simulink model "ControllerDesign_Lon"  (R2017b)
settings: Solver=VariableStepAuto  StartTime=0.0  StopTime=5  RelTol=1e-3
undefined symbols (not defined in the file or in its folder): Linmod
settings Model: Creator=One  LastModifiedBy=One

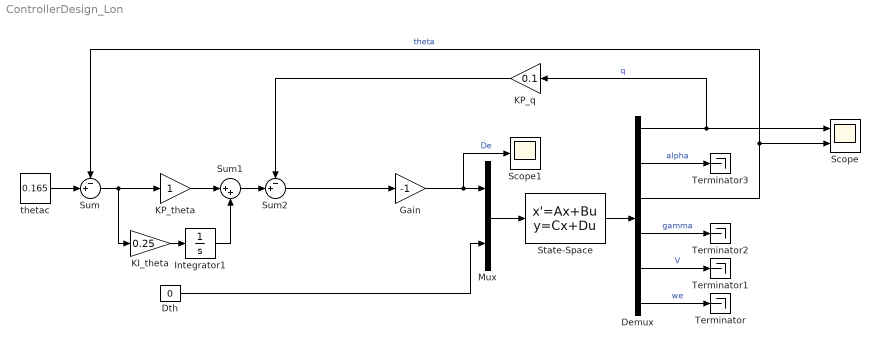
== system ControllerDesign_Lon ==
  Demux : Demux  Outputs=6
  Dth : Constant  Value=0  SampleTime=0.01
  Gain : Gain  Gain=-1
  Integrator1 : Integrator
  KI_theta : Gain  Gain=0.25
  KP_q : Gain  Gain=0.1
  KP_theta : Gain
  Mux : Mux  Inputs=2
  Scope : Scope  NumInputPorts=2
  Scope1 : Scope
  State-Space : StateSpace  A=Linmod.Lon_4b.A  B=Linmod.Lon_4b.B  C=Linmod.Lon_4b.C  D=Linmod.Lon_4b.D  InitialCondition=0
  Sum : Sum  Inputs=-+|
  Sum1 : Sum  Inputs=|++
  Sum2 : Sum  Inputs=-+|
  Terminator{,1..3} (4 alike) : Terminator
  thetac : Constant  Value=0.165  SampleTime=0.01
  wires:
  Mux/1 -> State-Space/1
  State-Space/1 -> Demux/1
  Dth/1 -> Mux/2
  Demux/6 -> Terminator/1  "we"
  Demux/5 -> Terminator1/1  "V"
  Demux/4 -> Terminator2/1  "gamma"
  Demux/2 -> Terminator3/1  "alpha"
  Demux/1 -> KP_q/1, Scope/1  "q"
  Demux/3 -> Scope/2, Sum/1  "theta"
  Gain/1 -> Scope1/1, Mux/1  "De"
  thetac/1 -> Sum/2
  Sum/1 -> KI_theta/1, KP_theta/1
  KI_theta/1 -> Integrator1/1
  KP_theta/1 -> Sum1/1
  Sum1/1 -> Sum2/2
  KP_q/1 -> Sum2/1
  Sum2/1 -> Gain/1
  Integrator1/1 -> Sum1/2
